simulink model "loadflowstudy"  (R2024b)
settings: Solver=ode23tb  StartTime=0.0  StopTime=10.0  MaxStep=1e-4  RelTol=1e-3
libraries: spsThreePhaseVIMeasurementLib x3, spsThreePhaseSeriesRLCBranchLib x3, spsLoadFlowBusLib x3, spsThreePhaseSourceLib x2, spsThreePhaseParallelRLCLoadLib x1, sps_lib x1
settings Model: Creator=brain  LastModifiedBy=brain

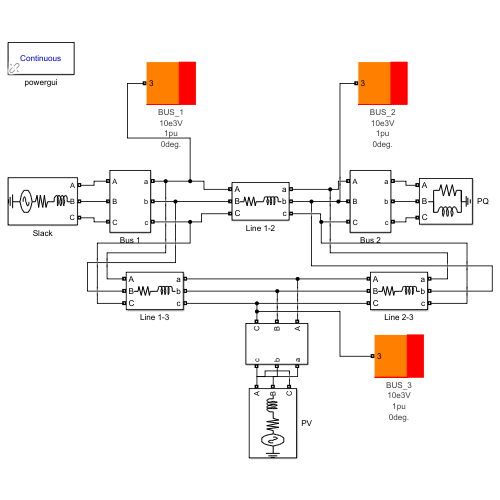
[thumbnail: Simulink's stored preview of the top-level diagram]
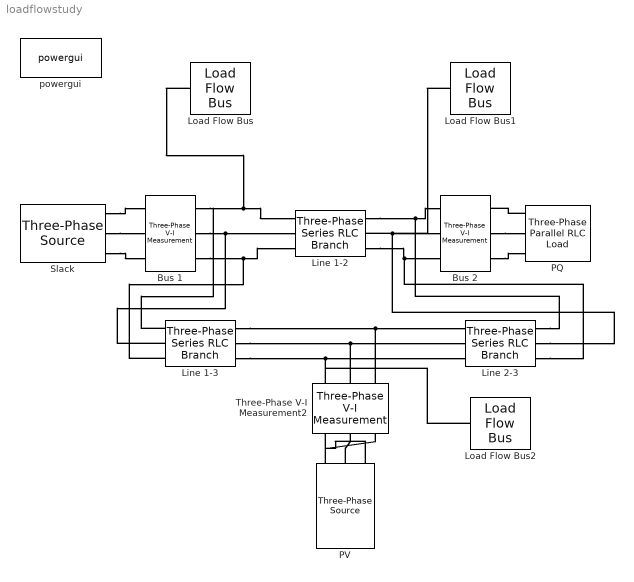
== system loadflowstudy ==
  Bus 1 : spsThreePhaseVIMeasurementLib/Three-Phase V-I Measurement  VoltageMeasurement=no  SetLabelV=off  LabelV=Vabc  Vpu=off  VpuLL=off  CurrentMeasurement=no  SetLabelI=off  LabelI=Iabc  Ipu=off  Pbase=100e6  Vbase=500e3  OutputType=Complex  PhasorSimulation=off  PSBequivalent=0
  Bus 2 : spsThreePhaseVIMeasurementLib/Three-Phase V-I Measurement  VoltageMeasurement=no  SetLabelV=off  LabelV=Vabc  Vpu=off  VpuLL=off  CurrentMeasurement=no  SetLabelI=off  LabelI=Iabc  Ipu=off  Pbase=100e6  Vbase=500e3  OutputType=Complex  PhasorSimulation=off  PSBequivalent=0
  Line 1-2 : spsThreePhaseSeriesRLCBranchLib/Three-Phase Series RLC Branch  LConnTagsString=A|B|C  RConnTagsString=A|B|C  BranchType=RL  Resistance=0.02  Inductance=0.04/(2*pi*60)  Capacitance=1e-6  Measurements=None
  Line 1-3 : spsThreePhaseSeriesRLCBranchLib/Three-Phase Series RLC Branch  LConnTagsString=A|B|C  RConnTagsString=A|B|C  BranchType=RL  Resistance=0.01  Inductance=0.03/(2*pi*60)  Capacitance=1e-6  Measurements=None
  Line 2-3 : spsThreePhaseSeriesRLCBranchLib/Three-Phase Series RLC Branch  LConnTagsString=A|B|C  RConnTagsString=A|B|C  BranchType=RL  Resistance=0.0125  Inductance=0.025/(2*pi*60)  Capacitance=1e-6  Measurements=None
  Load Flow Bus : spsLoadFlowBusLib/Load Flow Bus  LConnTagsString=a  Phases=single  Connectors=on one side  ID=BUS_1  Vbase=10e3  Vref=1.05  Vangle=0  VLF=1  VLFb=1  VLFc=1  angleLF=0  angleLFb=0  angleLFc=0
  Load Flow Bus1 : spsLoadFlowBusLib/Load Flow Bus  LConnTagsString=a  Phases=single  Connectors=on one side  ID=BUS_2  Vbase=10e3  Vref=1  Vangle=0  VLF=1  VLFb=1  VLFc=1  angleLF=0  angleLFb=0  angleLFc=0
  Load Flow Bus2 : spsLoadFlowBusLib/Load Flow Bus  LConnTagsString=a  Phases=single  Connectors=on one side  ID=BUS_3  Vbase=10e3  Vref=1.04  Vangle=0  VLF=1  VLFb=1  VLFc=1  angleLF=0  angleLFb=0  angleLFc=0
  PQ : spsThreePhaseParallelRLCLoadLib/Three-Phase Parallel RLC Load  LConnTagsString=A|B|C  Configuration=Y (grounded)  NominalVoltage=10e-3  Vabc=[1e3 1e3 1e3]  Vabcp=[1e3 1e3 1e3]  NominalFrequency=60  UnbalancedPower=off  ActivePower=190e6  InductivePower=250e6  CapacitivePower=0  Pabc=[10e3 9e3 11e3]  QLabc=[100 90 110]  QCabc=[100 90 110]  Pabcp=[10e3 9e3 11e3]  QLabcp=[100 90 110]  QCabcp=[100 90 110]  Measurements=None  LoadType=constant PQ
  PV : spsThreePhaseSourceLib/Three-Phase Source  InternalConnection=Yg  VoltagePhases=off  Voltage=10e3  PhaseAngle=0  Voltage_phases=[25e3 25e3 25e3]/sqrt(3)  PhaseAngles_phases=[0 -120 +120]  Frequency=60  NonIdealSource=on  SpecifyImpedance=off  Resistance=0.8929  Inductance=16.58e-3  ShortCircuitLevel=100e6  BaseVoltage=10e3  XRratio=7  BusType=PV  Pref=380  Qref=0  Prefabc=[10e3, 10e3, 10e3]  Qrefabc=[0, 0, 0]  Qmin=-inf  Qmax=inf
  Slack : spsThreePhaseSourceLib/Three-Phase Source  InternalConnection=Yg  VoltagePhases=off  Voltage=10e3  PhaseAngle=0  Voltage_phases=[25e3 25e3 25e3]/sqrt(3)  PhaseAngles_phases=[0 -120 +120]  Frequency=60  NonIdealSource=on  SpecifyImpedance=off  Resistance=0.8929  Inductance=16.58e-3  ShortCircuitLevel=100e6  BaseVoltage=10e3  XRratio=7  BusType=swing  Pref=10e3  Qref=0  Prefabc=[10e3, 10e3, 10e3]  Qrefabc=[0, 0, 0]  Qmin=-inf  Qmax=inf
  Three-Phase V-I Measurement2 : spsThreePhaseVIMeasurementLib/Three-Phase V-I Measurement  VoltageMeasurement=no  SetLabelV=off  LabelV=Vabc  Vpu=off  VpuLL=off  CurrentMeasurement=no  SetLabelI=off  LabelI=Iabc  Ipu=off  Pbase=100e6  Vbase=500e3  OutputType=Complex  PhasorSimulation=off  PSBequivalent=0
  powergui : sps_lib/powergui  Priority=1  SimulationMode=Continuous  SampleTime=50e-6  frequency=60  Iterations=50  frequencyindice=60  Pbase=100e6  ErrMax=1e-4  UnitsV=kV  UnitsW=MW  buscounter=0  FunctionMessages=off  echomessages=off  EnableUseOfTLC=off  CurrentSourceSwitches=off  DisableSnubberDevices=off  DisableRonSwitches=off  DisableVfSwitches=off  DisplayEquations=off  AutomaticDiscreteSolvers=off  SolverType=Tustin/Backward Euler (TBE)  Interpol=off  ExternalGateDelay=off  methode=off  Ts=100  x0status=blocks  SPID=on  SwTol=0  HookPort=off  NonlinearTolerance=1e-4  nMaxIteration=100  ContinueOnMaxIteration=off  RestoreLinks=warning  ResistiveCurrentMeasurement=off  Frange=[0:2:500]  Ylog=off  Xlog=on  ShowGrid=off  save=off  variable=ZData  structure=0  ZoomFFT=off  StartTime=0.0  cycles=1  DisplayStyle=1  fundamental=60  FreqAxis=off  MaxFrequency=1000  frequencyindicesteady=1  RmsSteady=1  display=off
  connections:
  Slack/RConn1 -- Bus 1/LConn1
  Slack/RConn2 -- Bus 1/LConn2
  Slack/RConn3 -- Bus 1/LConn3
  Line 1-3/RConn1 -- Three-Phase V-I Measurement2/LConn1 -- Line 2-3/LConn1
  Load Flow Bus1/LConn1 -- Bus 2/LConn2 -- Line 2-3/RConn2 -- Line 1-2/RConn2
  Bus 1/RConn3 -- Line 1-3/LConn3 -- Line 1-2/LConn3
  PQ/LConn1 -- Bus 2/RConn1
  Bus 2/RConn2 -- PQ/LConn2
  Bus 2/RConn3 -- PQ/LConn3
  Line 1-2/RConn3 -- Line 2-3/RConn3 -- Bus 2/LConn3
  Bus 1/RConn2 -- Line 1-3/LConn2 -- Line 1-2/LConn2
  Load Flow Bus/LConn1 -- Line 1-3/LConn1 -- Bus 1/RConn1 -- Line 1-2/LConn1
  PV/RConn1 -- Three-Phase V-I Measurement2/RConn1
  PV/RConn2 -- Three-Phase V-I Measurement2/RConn2
  PV/RConn3 -- Three-Phase V-I Measurement2/RConn3
  Line 1-3/RConn3 -- Load Flow Bus2/LConn1 -- Three-Phase V-I Measurement2/LConn3 -- Line 2-3/LConn3
  Line 1-3/RConn2 -- Three-Phase V-I Measurement2/LConn2 -- Line 2-3/LConn2
  Line 1-2/RConn1 -- Line 2-3/RConn1 -- Bus 2/LConn1
